simulink model "mech_flexible_cantilever"  (Simulink 7.1)
settings: Solver=ode15s  StartTime=0.0  StopTime=10  RelTol=5e-3
PreLoadFcn:
  | %-----------------------------------------
  | % Defined in the block mask
  | %-----------------------------------------
  | fBeamElement.material = 'Mild Steel';
  | 
  | % Beam element density (Kg/m^3)
  | fBeamElement.density = 7600;
  | 
  | fBeamElement.LengX = 1E-2;
  | fBeamElement.LengY = 1E-2;
  | 
  | % Beam element area of cross-section (m^2)
  | fBeamElement.crossArea = fBeamElement.LengX * fBeamElement.LengY;
  | 
  | % Beam element length (m)
  | fBeamElement.length = 0.15;
  | 
  | % Length of CG vector along length of beam (m)
  | fBeamElement.cgLeng = fBeamElement.length/2;
  | 
  | % Beam element direction (along X direction it is [1 0 0])
  | fBeamElement.beamDir = [1 0 0];
  | 
  | % Beam element Mass Moment of Inertia (Kg/m^2)
  | fBeamElement.Inertia = [120 0 0;0 6400.0 0;0 0 6400.0]*5E-8;
  | 
  | % Beam element Youngs Modulus (N/m^2)
  | fBeamElement.youngsM = 210E9;
  | 
  | % Beam element Shear Modulus (N/m^2)
  | fBeamElement.shearM = 26E9;
  | 
  | % Beam element Area Moment of Inertia along the direction of bending (m^4)
  | fBeamElement.Ixx = fBeamElement.LengX * fBeamElement.LengY^3/12;
  | 
  | % Beam element Area Moment of Inertia normal to the direction of
  | % bending (m^4)
  | fBeamElement.Iyy = fBeamElement.LengY * fBeamElement.LengX^3/12;
  | 
  | % Damping Coeff
  | fBeamElement.matDamping = 3.5;
  | %-----------------------------------------
InitFcn:
  | %-----------------------------------------
  | % Defined in the block mask
  | %-----------------------------------------
  | fBeamElement.material = 'Mild Steel';
  | 
  | % Beam element density (Kg/m^3)
  | fBeamElement.density = 7600;
  | 
  | fBeamElement.LengX = 1E-2;
  | fBeamElement.LengY = 1E-2;
  | 
  | % Beam element area of cross-section (m^2)
  | fBeamElement.crossArea = fBeamElement.LengX * fBeamElement.LengY;
  | 
  | % Beam element length (m)
  | fBeamElement.length = 0.15;
  | 
  | % Length of CG vector along length of beam (m)
  | fBeamElement.cgLeng = fBeamElement.length/2;
  | 
  | % Beam element direction (along X direction it is [1 0 0])
  | fBeamElement.beamDir = [1 0 0];
  | 
  | % Beam element Mass Moment of Inertia (Kg/m^2)
  | fBeamElement.Inertia = [120 0 0;0 6400.0 0;0 0 6400.0]*5E-8;
  | 
  | % Beam element Youngs Modulus (N/m^2)
  | fBeamElement.youngsM = 210E9;
  | 
  | % Beam element Shear Modulus (N/m^2)
  | fBeamElement.shearM = 26E9;
  | 
  | % Beam element Area Moment of Inertia along the direction of bending (m^4)
  | fBeamElement.Ixx = fBeamElement.LengX * fBeamElement.LengY^3/12;
  | 
  | % Beam element Area Moment of Inertia normal to the direction of
  | % bending (m^4)
  | fBeamElement.Iyy = fBeamElement.LengY * fBeamElement.LengX^3/12;
  | 
  | % Damping Coeff
  | fBeamElement.matDamping = 3.5;
  | %-----------------------------------------
libraries: mech_flexible_element_lib x10, mblibv1 x5
Description:
  | This demo illusatrates a cantilever flexing in one dimension
  | and modeled as a set of finite elements. This model uses
  | library blocks, data strcutures, and scripts to create and
  | configure multiple finite elements.
  | 
  | The tip of the cantilever is subjected to a load during part of
  | the simulation.  The entire cantilever is also subject
  | to its own weight in gravity.
  | 
  | 
  | Reference
  | 
  | Klaus-Jurgen Bathe, Finite Element Procedures, 1996 Prentice Hall Inc
  | 
  | Iakov Nakhimovski, Modeling and Simulation of Contacting Flexible Bodies in Multibody Systems,
  | Department of Computer and Information Science,
  | Lingoping University, Sweden, 2002, Thesis No 989.
settings Model: Creator=arnav  LastModifiedBy=batserve  ExtModeAutoUpdateStatusClock=off
settings SolverCC: MaxOrder=2
settings DebuggingCC: SaveWithParameterizedLinksMsg=none  SignalResolutionControl=TryResolveAllWithWarning  SolverPrmCheckMsg=none  MultiTaskDSMMsg=warning  MultiTaskCondExecSysMsg=none  SigSpecEnsureSampleTimeMsg=none  StrictBusMsg=None
settings HardwareCC: TargetBitPerLong=64  TargetEndianess=LittleEndian  TargetWordSize=64  TargetHWDeviceType=MATLAB Host  ProdEqTarget=off
settings RTWCC: SystemTargetFile=rsim.tlc  TemplateMakefile=rsim_default_tmf  Description=Rapid Simulation Target  ProcessScript=rsim_make_rtw_hook  IncludeERTFirstTime=on
settings RSimTargetCC: TargetFcnLib=ansi_tfl_tmw.mat  TargetFunctionLibrary=ANSI_C  IsPILTarget=off  EnableShiftOperators=on  PortableWordSizes=off
settings SimMechanicsCC: WarnOnRedundantConstraints=off  VisOnUpdateDiagram=on  VisDuringSimulation=on  VisConfigFile=mech_flexible_cantilever.mat

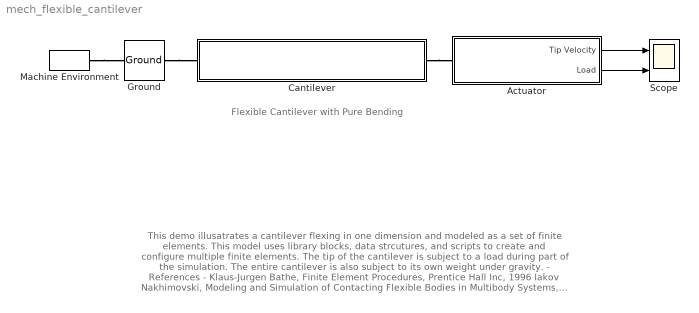
== system mech_flexible_cantilever ==
  note: Flexible Cantilever with Pure Bending
  note: This demo illusatrates a cantilever flexing in one dimension
      | and modeled as a set of finite elements. This model uses
      | library blocks, data strcutures, and scripts to create and
      | configure multiple finite elements.
      |
      | The tip of the cantilever is subject to a load during part of
      | the simulation.  The entire cantilever is also subject
      | to its own weight under gravity.
      |
      | - References -
      |
      | Klaus-Jurgen Bathe, Finite Element Procedures, Prentice Hall Inc, 1996
      |
      | Iakov Nakhimovski, Modeling and Simulation of Contacting Flexible Bodies in Multibody Systems,
      | Department of Computer and Information Science,
      | Lingoping University, Sweden, 2002, Thesis No 989
  Actuator : Subsystem
  Cantilever : Subsystem
  Ground : mblibv1/Bodies/Ground  DialogController=MECH.DynMechDlgSource  SystemSampleTime=-1  LeftPortType=env  RightPortType=workingframe  PhysicalDomain=Mechanical  DialogClass=GroundBlock  CoordPosition=[0 0 0]  CoordPositionUnits=m  StateVectorMgrId=-1  MachineId=[0 0]  ShowEnvPort=on
  Machine Environment : mblibv1/Bodies/Machine Environment  Tag=Factory ground  DialogController=MECH.DialogSource  SystemSampleTime=-1  PortType=env  PhysicalDomain=Mechanical  DialogTemplateClass=MECH.MachineEnvironment  SyncWhenCopied=off  Gravity=[0 -9.81 0]  GravityUnits=m/s^2  GravityAsSignal=off  Dimensionality=Auto-detect  AnalysisType=Forward dynamics  LinearAssemblyTolerance=1e-3  LinearAssemblyToleranceUnits=m  AngularAssemblyTolerance=1e-3  AngularAssemblyToleranceUnits=rad  ConstraintSolverType=Stabilizing  ConstraintRelTolerance=1e-4  ConstraintAbsTolerance=1e-4  UseRobustSingularityHandling=off  RedundancyAnalysisToleranceType=Automatically select tolerance  RedundancyAnalysisTolerance=1e-14  StatePerturbationType=Fixed  PerturbationSize=1e-5  VisualizeMachine=on
  Scope : Scope  NumInputPorts=2
      settings: TimeRange=10  YMin=-10~-60  YMax=10~10
  wires:
  Actuator/1(Tip Velocity) -> Scope/1
  Actuator/2(Load) -> Scope/2
  connections:
  Machine Environment/RConn1 -- Ground/LConn1
  Ground/RConn1 -- Cantilever/LConn1
  Cantilever/RConn1 -- Actuator/LConn1

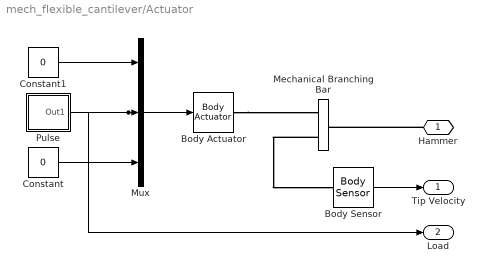
== system mech_flexible_cantilever/Actuator ==
  Body Actuator : mblibv1/Sensors &  Actuators/Body Actuator  DialogController=MECH.DynMechDlgSource  SystemSampleTime=-1  PhysicalDomain=Mechanical  PortType=blob  ActuationStyle=Force  AngleUnits=deg  ArcVelocityUnits=deg/s  ArcAccelerationUnits=deg/s^2  CoordPositionUnits=m  VelocityUnits=m/s  AccelerationUnits=m/s^2  ForceUnits=N  TorqueUnits=N-m  ActiveIO=on  Width=3  DialogClass=MechanicalActuatorBlock  ReferenceFrame=Absolute (World)  Angle=off  CoordPosition=on  Force=on  Torque=off
  Body Sensor : mblibv1/Sensors &  Actuators/Body Sensor  DialogController=MECH.DynMechDlgSource  SystemSampleTime=-1  PhysicalDomain=Mechanical  PortType=blob  Muxed=on  Pose=off  Angle=on  AngleUnits=deg  ArcVelocity=on  ArcVelocityUnits=rad/s  ArcAcceleration=off  ArcAccelerationUnits=deg/s^2  CoordPosition=off  CoordPositionUnits=m  Velocity=off  VelocityUnits=m/s  Acceleration=off  AccelerationUnits=m/s^2  Quaternion=on  QuaternionDT=off  QuaternionDDT=off  QuaternionUnits=off  OutputVector=[ 3 ]  ActiveIO=on  Width=3  DialogClass=MechanicalSensorBlock  ReferenceFrame=Absolute (World)
  Constant : Constant  Value=0  OutDataType=sfix(16)  OutScaling=2^0
  Constant1 : Constant  Value=0  OutDataType=sfix(16)  OutScaling=2^0
  Mechanical Branching Bar : mblibv1/Utilities/Mechanical Branching Bar  Orientation=left  DialogController=MECH.DynMechDlgSource  PhysicalDomain=mechanical  SubClassName=Unknown  LeftPortType=blob  RightPortType=blob  LConnTagsString=_newl0  RConnTagsString=SA0|SA1  DialogClass=MechanicalBranchingBarBlock  NumSAPorts=2
  Mux : Mux  Inputs=3
  Pulse : Subsystem
  Hammer : PMIOPort  Orientation=left  Port=1  Side=Left
  Tip Velocity : Outport  OutDataType=sfix(16)  OutScaling=2^0
  Load : Outport  Port=2  OutDataType=sfix(16)  OutScaling=2^0
  wires:
  Constant1/1 -> Mux/1
  Constant/1 -> Mux/3
  Mux/1 -> Body Actuator/1
  Pulse/1(Out1) -> Mux/2, Load/1
  Body Sensor/1 -> Tip Velocity/1
  connections:
  Body Actuator/RConn1 -- Mechanical Branching Bar/RConn1
  Mechanical Branching Bar/RConn2 -- Body Sensor/LConn1
  Hammer/RConn1 -- Mechanical Branching Bar/LConn1

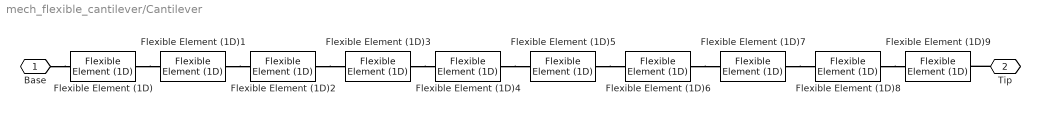
== system mech_flexible_cantilever/Cantilever ==
  Flexible Element (1D){,1..9} (10 alike) : mech_flexible_element_lib/Flexible Element (1D)  SystemSampleTime=-1  material=Mild Steel  density=fBeamElement.density  crossArea=fBeamElement.crossArea  length=fBeamElement.length  cgLeng=fBeamElement.cgLeng  beamDir=fBeamElement.beamDir  Inertia=fBeamElement.Inertia  youngsM=fBeamElement.youngsM  shearM=26E9  Ixx=fBeamElement.Ixx  Iyy=8.3333e-010  matDamping=fBeamElement.matDamping
  Base : PMIOPort  Port=1  Side=Left
  Tip : PMIOPort  Orientation=left  Port=2  Side=Right
  connections:
  Tip/RConn1 -- Flexible Element (1D)9/RConn1
  Base/RConn1 -- Flexible Element (1D)/LConn1
  Flexible Element (1D)/RConn1 -- Flexible Element (1D)1/LConn1
  Flexible Element (1D)1/RConn1 -- Flexible Element (1D)2/LConn1
  Flexible Element (1D)2/RConn1 -- Flexible Element (1D)3/LConn1
  Flexible Element (1D)3/RConn1 -- Flexible Element (1D)4/LConn1
  Flexible Element (1D)4/RConn1 -- Flexible Element (1D)5/LConn1
  Flexible Element (1D)5/RConn1 -- Flexible Element (1D)6/LConn1
  Flexible Element (1D)6/RConn1 -- Flexible Element (1D)7/LConn1
  Flexible Element (1D)7/RConn1 -- Flexible Element (1D)8/LConn1
  Flexible Element (1D)8/RConn1 -- Flexible Element (1D)9/LConn1

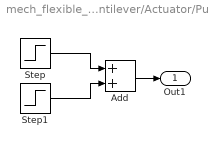
== system mech_flexible_cantilever/Actuator/Pulse ==
  Add : Sum  OutDataType=sfix(16)  OutScaling=2^-10
  Step : Step  Time=4  Before=-50  After=0  SampleTime=0
  Step1 : Step  Time=0.5  Before=50  After=0  SampleTime=0
  Out1 : Outport  OutDataType=sfix(16)  OutScaling=2^0
  wires:
  Add/1 -> Out1/1
  Step1/1 -> Add/2
  Step/1 -> Add/1
